simulink model "EngineControl_SLPV"  (R2016b)
settings: Solver=ode23tb  StartTime=0.0  StopTime=60  FixedStep=1e-3  MaxStep=1e-2  RelTol=0.001  EnableMultiTasking=on
values from neighbouring files (symbols this model uses):
  alpha = 0.1    [main_slpv.m]
  Ap = plt.a    [plant_sel.m]
  Bp = plt.b    [plant_sel.m]
  Cp = plt.c    [plant_sel.m]
  Dp = plt.d    [plant_sel.m]
  swtch = 1    [main_slpv.m]
  Wi = ss(tf([0.6 2],[1 0]))    [plant_sel.m]
undefined symbols (not defined in the file or in its folder): Khinf, sigbuilder_block
undefined symbols (not defined in the file): design_para, Dk, OptRst, theta_info
libraries: simulink x3
settings Model: Creator=Marius  LastModifiedBy=boran
settings DataIOCC: LimitDataPoints=on  SaveFormat=Array  SignalLoggingSaveFormat=ModelDataLogs
settings OptimizationCC: ExpressionDepthLimit=2147483647  InitFltsAndDblsToZero=on  LifeSpan=inf
settings DebuggingCC: UnderspecifiedInitializationDetection=Classic  MergeDetectMultiDrivingBlocksExec=none  SolverPrmCheckMsg=warning  FcnCallInpInsideContextMsg=warning  AllowSymbolicDim=off  StateNameClashWarn=warning  SFUnexpectedBacktrackingDiag=warning  SFNoUnconditionalDefaultTransitionDiag=warning  SFExecutionAtInitializationDiag=none
settings HardwareCC: ProdBitPerPointer=32  ProdBitPerSizeT=32  ProdBitPerPtrDiffT=32  ProdLargestAtomicFloat=None  ProdIntDivRoundTo=Undefined  ProdEndianess=Unspecified  ProdWordSize=32  ProdHWDeviceType=32-bit Generic
settings ModelReferenceCC: PropagateSignalLabelsOutOfModel=off
settings SFSimCC: SimParseCustomCode=off
settings GRTTargetCC: TargetLangStandard=C89/C90 (ANSI)  CombineOutputUpdateFcns=off  GRTInterface=on
settings ConfigComp: CovMetricSettings=dw  CovHtmlReporting=on  CovSaveCumulativeToWorkspaceVar=on  CovSaveSingleToWorkspaceVar=on  CovExternalEMLEnable=off  CovSFcnEnable=off

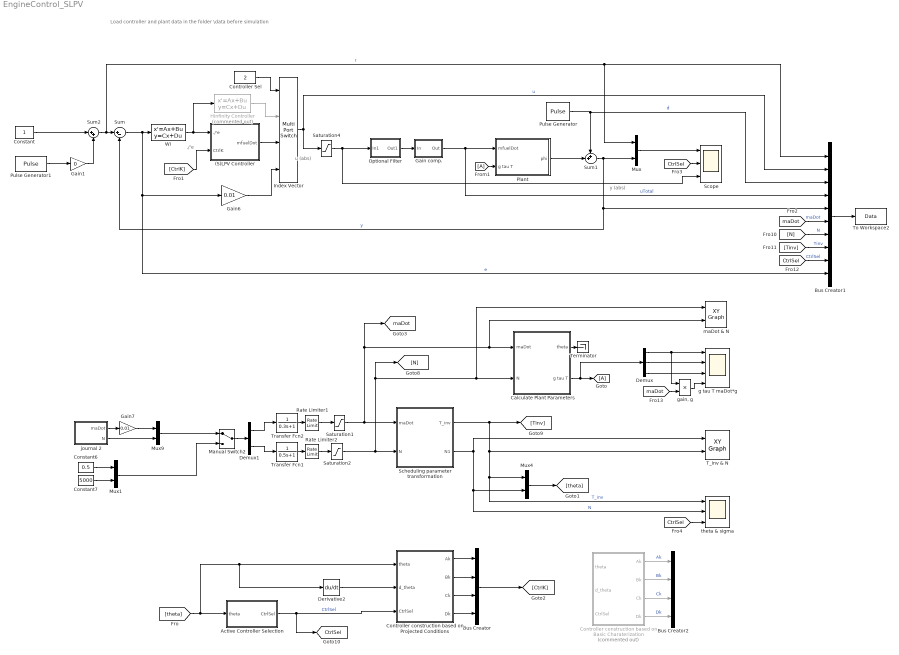
== system EngineControl_SLPV ==
  note: Load controller and plant data in the folder \data before simulation
  note: y (abs)
  note: u (abs)
  note: ./'e
  "(S)LPV Controller " : Subsystem
  Active Controller Selection : Subsystem
  Bus Creator : BusCreator  Inputs=4
  Bus Creator1 : BusCreator  Inputs=10
  Bus Creator2 : BusCreator  Inputs=4
  Calculate Plant Parameters : Subsystem
  Constant : Constant
  Constant6 : Constant  Value=0.5
  Constant7 : Constant  Value=5000
  Controller Sel : Constant  Value=2
  Controller construction based on Basic Charaterization : MATLAB Function  Commented=on  TreatAsAtomicUnit=on  mask{XY_PD=design_para.XY_PD, X=OptRst.X, Y=OptRst.Y, Ah=OptRst.K.Ah, Bh=OptRst.K.Bh, Ch=OptRst.K.Ch, Dh=OptRst.K.Dh, B2=0, C2=0}
  Controller construction based on Projected Conditions : MATLAB Function  TreatAsAtomicUnit=on  mask{XY_PD=design_para.XY_PD, X=OptRst.X, Y=OptRst.Y, Dk1=Dk, gam=OptRst.gam}
      mask prompts: Dk1 "Dk"
  Demux : Demux  Outputs=3
  Demux1 : Demux  Outputs=2
  Derivative2 : Derivative
  Gain comp. : Subsystem
  Gain1 : Gain  Gain=0
  Gain6 : Gain  Gain=0.01
  Gain7 : Gain  Gain=0.01
  Hinfinity Controller : StateSpace  Commented=on  A=Khinf.a  B=Khinf.b  C=Khinf.c  D=Khinf.d  X0=0
  Index Vector : MultiPortSwitch
  Manual Switch2 : ManualSwitch
  Mux{,1,4,9} (4 alike) : Mux  Inputs=2
  Optional Filter : Subsystem
  Plant : Subsystem
  Pulse Generator : DiscretePulseGenerator  PulseType=Time based  Amplitude=0.1  Period=20  PulseWidth=50
  Pulse Generator1 : DiscretePulseGenerator  PulseType=Time based  Amplitude=0.1  Period=20  PulseWidth=50
  Rate Limiter1 : RateLimiter
  Rate Limiter2 : RateLimiter  RisingSlewLimit=2000  FallingSlewLimit=-2000
  Saturation1 : Saturate  UpperLimit=1  LowerLimit=0.1  ZeroCross=off
  Saturation2 : Saturate  UpperLimit=6000  LowerLimit=800  ZeroCross=off
  Saturation4 : Saturate  UpperLimit=1  LowerLimit=0  ZeroCross=off
  Scheduling parameter transformation : Subsystem
  Scope : Scope  NumInputPorts=3
  Sum : Sum  Inputs=|+-
  Sum1 : Sum  Inputs=++|
  Sum2 : Sum  Inputs=|++
  T_inv & N : simulink/Sinks/XY Graph  xmin=0  xmax=6000  ymin=0  ymax=15  st=-1
  Terminator : Terminator
  To Workspace2 : ToWorkspace  VariableName=Data  SaveFormat=Timeseries  SampleTime=-1
  Transfer Fcn1 : TransferFcn  Denominator=[0.5 1]
  Transfer Fcn2 : TransferFcn  Denominator=[0.3 1]
  Wi : StateSpace  A=Wi.a  B=Wi.b  C=Wi.c  D=Wi.d  X0=0
  g tau T maDot*g : Scope  NumInputPorts=4
  "gain, g" : Product  RndMeth=Zero
  journal 2 : Subsystem  Tag=STV Subsys  LoadFcn=sigbuilder_block('load');  StartFcn=sigbuilder_block('start');  StopFcn=sigbuilder_block('stop');  ClipboardFcn=sigbuilder_block('clipboard');  mask(Sigbuilder block){tuvar=[0:10]}
      mask help: Sigbuilder GUI
      mask init:
      | if ~strcmp(get_param(bdroot(gcbh),'SimulationStatus'),'stopped') tuvar = sigbuilder_block('maskInit'); end
      settings: CopyFcn=sigbuilder_block('copy');  DeleteFcn=sigbuilder_block('delete');  ModelCloseFcn=sigbuilder_block('modelClose');  PreSaveFcn=sigbuilder_block('preSave');  PauseFcn=sigbuilder_block('pause')  ContinueFcn=sigbuilder_block('continue')  NameChangeFcn=sigbuilder_block('namechange');  OpenFcn=sigbuilder_block('open',[-1117.5 98.25 1428 499.5 ]);  CloseFcn=sigbuilder_block('close');
      mask Display: plot(0,0,100,100,[10,10,40,40,10],[80,20,20,80,80],[40,10],[50,50], [40,27,10],[65,72,56],[40,25,25,10],[28,28,43,43]);
  maDot & N : simulink/Sinks/XY Graph  xmin=0  xmax=6000  ymin=0  ymax=1  st=-1
  theta & sigma : Scope  NumInputPorts=3
  tag scope: CtrlSel=global, maDot=global
  wires:
  Mux/1 -> Scope/1
  Sum1/1 -> Mux/2, Bus Creator1/5, Sum/2  "y"
  Constant/1 -> Sum2/1
  Calculate Plant Parameters/1(theta) -> Terminator/1
  Demux/1 -> "gain, g"/1, g tau T maDot*g/1
  Demux/2 -> g tau T maDot*g/2
  Demux/3 -> g tau T maDot*g/3
  Calculate Plant Parameters/2(g tau T) -> [A], Demux/1
  [A] -> Plant/2(g tau T)
  Scheduling parameter transformation/2(N1) -> Mux4/2, theta & sigma/2, T_inv & N/1  "N"
  Scheduling parameter transformation/1(T_inv) -> T_inv & N/2, theta & sigma/1, Mux4/1, [Tinv]  "T_inv"
  Rate Limiter2/1 -> Saturation2/1
  Mux4/1 -> [theta]
  [theta] -> Derivative2/1, Controller construction based on Projected Conditions/1(theta), Active Controller Selection/1(theta)
  Controller construction based on Projected Conditions/3(Ck) -> Bus Creator/3
  Controller construction based on Projected Conditions/2(Bk) -> Bus Creator/2
  Controller construction based on Projected Conditions/4(Dk) -> Bus Creator/4
  Controller construction based on Projected Conditions/1(Ak) -> Bus Creator/1
  Active Controller Selection/1(CtrlSel) -> [CtrlSel], Controller construction based on Projected Conditions/3(CtrlSel)  "CtrlSel"
  Derivative2/1 -> Controller construction based on Projected Conditions/2(d_theta)
  Rate Limiter1/1 -> Saturation1/1
  Saturation1/1 -> Calculate Plant Parameters/1(maDot), maDot & N/2, [maDot], Scheduling parameter transformation/1(maDot)
  Mux1/1 -> Manual Switch2/2
  Plant/1(phi) -> Sum1/2
  Optional Filter/1(Out1) -> Gain comp./1(In)
  "(S)LPV Controller "/1(mfuelDot) -> Index Vector/3
  Hinfinity Controller/1 -> Index Vector/2
  Gain6/1 -> Index Vector/4
  Controller Sel/1 -> Index Vector/1
  Constant6/1 -> Mux1/1
  Constant7/1 -> Mux1/2
  Manual Switch2/1 -> Demux1/1
  Bus Creator1/1 -> To Workspace2/1
  Sum2/1 -> Sum/1, Mux/1, Bus Creator1/1  "r"
  Pulse Generator/1 -> Bus Creator1/3, Sum1/1  "d"
  Gain comp./1(Out) -> Bus Creator1/4, Plant/1(mfuelDot)  "uTotal"
  Index Vector/1 -> Saturation4/1, Bus Creator1/2  "u"
  [maDot] -> Bus Creator1/6  "maDot"
  [N] -> Bus Creator1/7  "N"
  [Tinv] -> Bus Creator1/8  "Tinv"
  [CtrlSel] -> Bus Creator1/9  "CtrlSel"
  Controller construction based on Basic Charaterization/1(Ak) -> Bus Creator2/1  "Ak"
  Controller construction based on Basic Charaterization/2(Bk) -> Bus Creator2/2  "Bk"
  Controller construction based on Basic Charaterization/3(Ck) -> Bus Creator2/3  "Ck"
  Controller construction based on Basic Charaterization/4(Dk) -> Bus Creator2/4  "Dk"
  [maDot] -> "gain, g"/2
  "gain, g"/1 -> g tau T maDot*g/4
  Bus Creator/1 -> [CtrlK]
  [CtrlK] -> "(S)LPV Controller "/2(CtrlK)
  Gain7/1 -> Mux9/1
  Mux9/1 -> Manual Switch2/1
  Saturation2/1 -> Calculate Plant Parameters/2(N), maDot & N/1, [N], Scheduling parameter transformation/2(N)
  Sum/1 -> Wi/1, Gain6/1, Bus Creator1/10  "e"
  Demux1/1 -> Transfer Fcn2/1
  Demux1/2 -> Transfer Fcn1/1
  Transfer Fcn2/1 -> Rate Limiter1/1
  Transfer Fcn1/1 -> Rate Limiter2/1
  journal 2/2(N) -> Mux9/2
  journal 2/1(maDot) -> Gain7/1
  Wi/1 -> "(S)LPV Controller "/1(./'e), Hinfinity Controller/1
  Saturation4/1 -> Optional Filter/1(In1), Scope/3
  Pulse Generator1/1 -> Gain1/1
  Gain1/1 -> Sum2/2
  [CtrlSel] -> Scope/2
  [CtrlSel] -> theta & sigma/3

== system EngineControl_SLPV/(S)LPV Controller  ==
  ./'e : Inport
  CtrlK : Inport  Port=2
  Controller2 : Subsystem
  Terminator1 : Terminator
  mfuelDot : Outport
  wires:
  Controller2/1(delta_u) -> mfuelDot/1
  Controller2/2(xk) -> Terminator1/1
  CtrlK/1 -> Controller2/2(CtrlK)
  ./'e/1 -> Controller2/1(./`e)

== system EngineControl_SLPV/Active Controller Selection ==
  theta : Inport
  Clock : Clock
  MATLAB Function2 : MATLAB Function  TreatAsAtomicUnit=on  mask{Theta1=theta_info.Theta1, Theta2=theta_info.Theta2, SwLogic=design_para.SwLogic, REGID=design_para.REGID}
  Memory1 : Memory  X0=1
  CtrlSel : Outport
  wires:
  theta/1 -> MATLAB Function2/1(theta)
  Memory1/1 -> MATLAB Function2/3(CtrlSel_t_1)
  MATLAB Function2/1(CtrlSel) -> CtrlSel/1, Memory1/1
  Clock/1 -> MATLAB Function2/2(time)

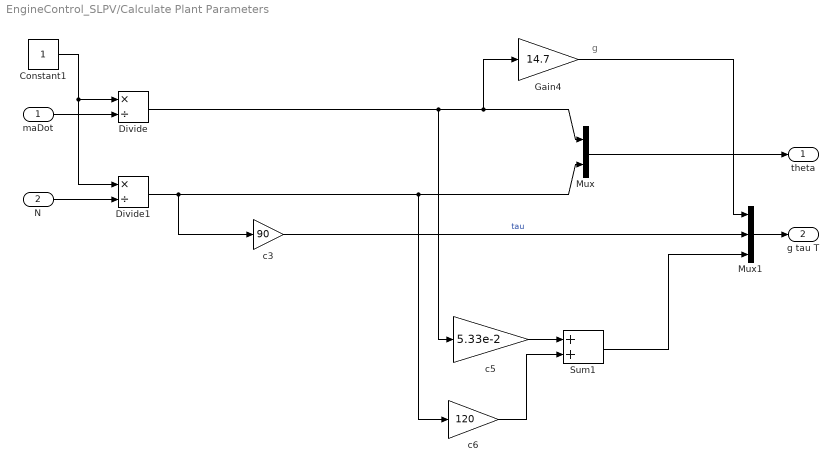
== system EngineControl_SLPV/Calculate Plant Parameters ==
  note: g
  maDot : Inport
  N : Inport  Port=2
  Constant1 : Constant
  Divide : Product  Inputs=*/
  Divide1 : Product  Inputs=*/
  Gain4 : Gain  Gain=14.7
  Mux : Mux  Inputs=2
  Mux1 : Mux  Inputs=3
  Sum1 : Sum
  c3 : Gain  Gain=90
  c5 : Gain  Gain=5.33e-2
  c6 : Gain  Gain=120
  theta : Outport
  g tau T : Outport  Port=2
  wires:
  Constant1/1 -> Divide/1, Divide1/1
  maDot/1 -> Divide/2
  N/1 -> Divide1/2
  Divide/1 -> c5/1, Gain4/1, Mux/1
  Divide1/1 -> c3/1, c6/1, Mux/2
  c6/1 -> Sum1/2
  c3/1 -> Mux1/2  "tau"
  Gain4/1 -> Mux1/1
  Mux/1 -> theta/1
  Mux1/1 -> g tau T/1
  c5/1 -> Sum1/1
  Sum1/1 -> Mux1/3

== system EngineControl_SLPV/Gain comp. ==
  In : Inport
  "gain, g" : Product  RndMeth=Zero
  Out : Outport
  wires:
  "gain, g"/1 -> Out/1
  [maDot] -> "gain, g"/2
  In/1 -> "gain, g"/1

== system EngineControl_SLPV/Optional Filter ==
  In1 : Inport
  Constant : Constant  Value=swtch+1
  Multiport Switch : MultiPortSwitch  Inputs=2
  Transfer Fcn : TransferFcn  Denominator=[alpha 1]
  Out1 : Outport
  wires:
  Multiport Switch/1 -> Out1/1
  In1/1 -> Transfer Fcn/1, Multiport Switch/2
  Transfer Fcn/1 -> Multiport Switch/3
  Constant/1 -> Multiport Switch/1

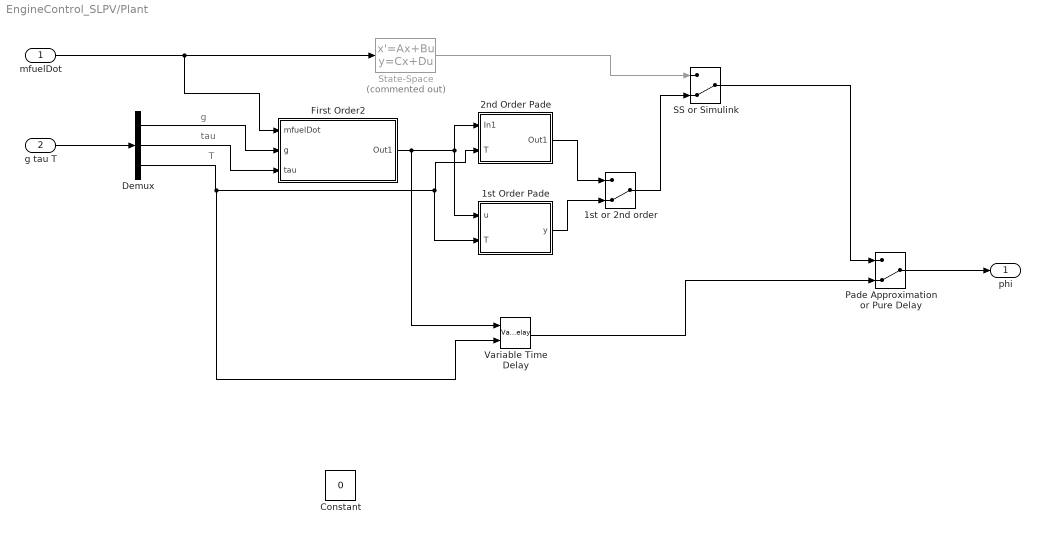
== system EngineControl_SLPV/Plant ==
  note: g
  note: tau
  note: T
  mfuelDot : Inport
  g tau T : Inport  Port=2
  1st Order Pade : Subsystem
  1st or 2nd order : ManualSwitch  CurrentSetting=0
  2nd Order Pade : Subsystem
  Constant : Constant  Value=0
  Demux : Demux  Outputs=3
  First Order2 : Subsystem
  Pade Approximation or Pure Delay : ManualSwitch  CurrentSetting=0
  SS or Simulink : ManualSwitch  CurrentSetting=0
  State-Space : StateSpace  Commented=on  A=Ap  B=Bp  C=Cp  D=Dp  X0=0
  Variable Time Delay : VariableTransportDelay  MaximumDelay=10  MaximumPoints=2048  ZeroDelay=on
  phi : Outport
  wires:
  Demux/1 -> First Order2/2(g)
  Demux/2 -> First Order2/3(tau)
  State-Space/1 -> SS or Simulink/1
  SS or Simulink/1 -> Pade Approximation or Pure Delay/1
  Pade Approximation or Pure Delay/1 -> phi/1
  g tau T/1 -> Demux/1
  2nd Order Pade/1(Out1) -> 1st or 2nd order/1
  1st Order Pade/1(y) -> 1st or 2nd order/2
  First Order2/1(Out1) -> Variable Time Delay/1, 2nd Order Pade/1(In1), 1st Order Pade/1(u)
  1st or 2nd order/1 -> SS or Simulink/2
  Variable Time Delay/1 -> Pade Approximation or Pure Delay/2
  mfuelDot/1 -> First Order2/1(mfuelDot), State-Space/1
  Demux/3 -> 2nd Order Pade/2(T), 1st Order Pade/2(T), Variable Time Delay/2

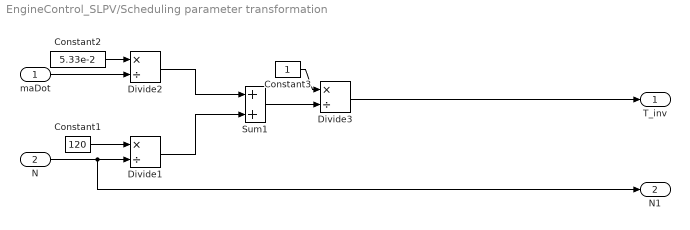
== system EngineControl_SLPV/Scheduling parameter transformation ==
  maDot : Inport
  N : Inport  Port=2
  Constant1 : Constant  Value=120
  Constant2 : Constant  Value=5.33e-2
  Constant3 : Constant
  Divide1 : Product  Inputs=*/
  Divide2 : Product  Inputs=*/
  Divide3 : Product  Inputs=*/
  Sum1 : Sum
  T_inv : Outport
  N1 : Outport  Port=2
  wires:
  N/1 -> N1/1, Divide1/2
  maDot/1 -> Divide2/2
  Constant1/1 -> Divide1/1
  Constant2/1 -> Divide2/1
  Divide2/1 -> Sum1/1
  Divide1/1 -> Sum1/2
  Sum1/1 -> Divide3/2
  Constant3/1 -> Divide3/1
  Divide3/1 -> T_inv/1

== system EngineControl_SLPV/journal 2 ==
  Demux : Demux  Tag=STV Demux  Outputs=2
  FromWs : FromWorkspace  Tag=STV FromWs  VariableName=tuvar  SampleTime=0
      SigBuilderData=|
      | common.afterFinalStr = 'Extrapolate'
      | common.sampleTime = 0
      | dataSet.timeRange = [0 90]
      | dataSet.name = 'Group 1'
      | sbobj.Groups.Name = 'Group 1'
      | sbobj.Groups.Signals(1).Name = 'maDot'
      | sbobj.Groups.Signals(1).XData = [0 3 5.6 8 10.9 14.8 19.7 22 24 26 27 30.8 32.5 33.5 35 36.2 38 39 39 41 41 43.4 45.5 47 48 52.3 54 56.5 59 60 65 65 70 90]
      | sbobj.Groups.Signals(1).YData = [10 10 13.6 13.5 19.1 38.6 39.1 26.6 29.1 65.1 97.6 98.6 98.6 40.6 40.6 96.6 97.1 97.1 97 96.5 97 45.1 81.1 82.1 40.1 40.6 63 38 33.5 33.5 35.5 40.1 39.1 8.5]
      | sbobj.Groups.Signals(2).Name = 'N'
      | sbobj.Groups.Signals(2).XData = [0 3 5.6 8 11.4 14 17 19.9 23 24 26.9 29 33.3 34.5 35.5 36.5 38 39 41 43.4 45.8 47.2 49 52 54 56.5 59 60 90]
      | sbobj.Groups.Signals(2).YData = [800 800 1000 800 1000 2050 5500 5500 2050 2000 2350 5750 5800 2620 2650 4850 4850 3700 3750 2750 3700 3700 2400 2400 3250 1800 1550 1550 1300]
      | sbobj.Groups.TimeRange = [0 90]
  maDot : Outport  Tag=STV Outport
  N : Outport  Tag=STV Outport  Port=2
  wires:
  FromWs/1 -> Demux/1
  Demux/1 -> maDot/1
  Demux/2 -> N/1

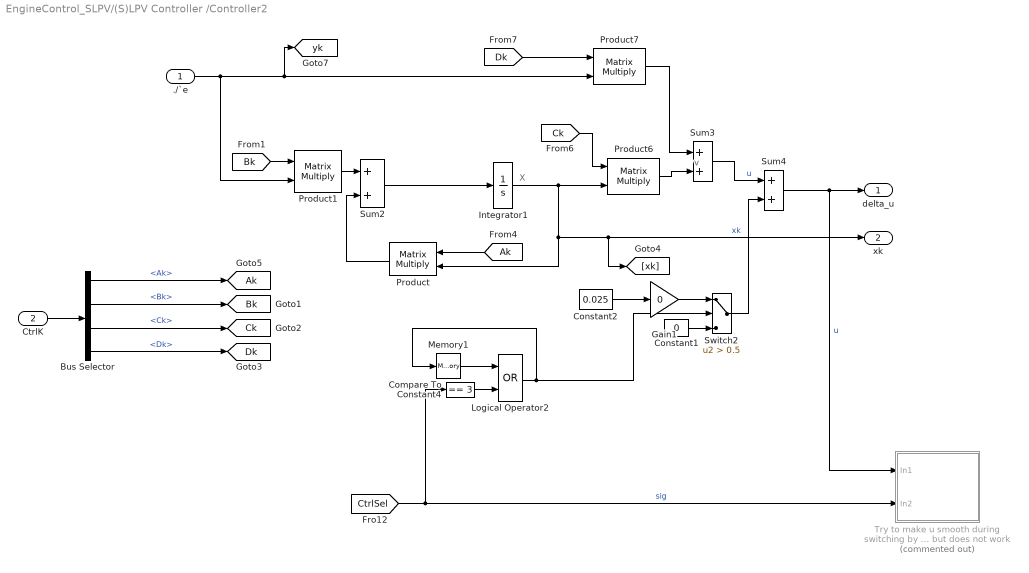
== system EngineControl_SLPV/(S)LPV Controller /Controller2 ==
  note: X
  note: v
  ./`e : Inport
  CtrlK : Inport  Port=2
  Bus Selector : BusSelector  OutputSignals=Ak,Bk,Ck,Dk
  Compare To Constant4 : simulink/Logic and Bit Operations/Compare To Constant  relop===  const=3  OutDataTypeStr=uint8
  Constant1 : Constant  Value=0
  Constant2 : Constant  Value=0.025  VectorParams1D=off
  Gain1 : Gain  Gain=0
  Integrator1 : Integrator
  Logical Operator2 : Logic  Operator=OR  AllPortsSameDT=off  OutDataTypeStr=boolean
  Memory1 : Memory
  Product{,1,6..7} (4 alike) : Product  Multiplication=Matrix(*)
  Sum2 : Sum
  Sum3 : Sum
  Sum4 : Sum
  Switch2 : Switch  Criteria=u2 > Threshold  Threshold=0.5
  Try to make u smooth during switching by resetting controller state but does not work : Subsystem  Commented=on
  delta_u : Outport
  xk : Outport  Port=2
  tag scope: Ak=global, Bk=global, Ck=global, Dk=global, yk=global
  wires:
  Sum4/1 -> Try to make u smooth during switching by resetting controller state but does not work/1(In1), delta_u/1  "u"
  [CtrlSel] -> Try to make u smooth during switching by resetting controller state but does not work/2(In2), Compare To Constant4/1  "sig"
  Product6/1 -> Sum3/2
  Product1/1 -> Sum2/1
  [Bk] -> Product1/1
  Product/1 -> Sum2/2
  [Ak] -> Product/1
  Bus Selector/4 -> [Dk]  "<Dk>"
  Bus Selector/3 -> [Ck]  "<Ck>"
  Bus Selector/2 -> [Bk]  "<Bk>"
  Bus Selector/1 -> [Ak]  "<Ak>"
  [Ck] -> Product6/1
  [Dk] -> Product7/1
  Product7/1 -> Sum3/1
  ./`e/1 -> Product1/2, Product7/2, [yk]
  Integrator1/1 -> Product/2, [xk], xk/1, Product6/2  "xk"
  Sum2/1 -> Integrator1/1
  CtrlK/1 -> Bus Selector/1
  Constant1/1 -> Switch2/3
  Logical Operator2/1 -> Switch2/2, Memory1/1
  Sum3/1 -> Sum4/1  "u"
  Switch2/1 -> Sum4/2
  Constant2/1 -> Gain1/1
  Compare To Constant4/1 -> Logical Operator2/2
  Memory1/1 -> Logical Operator2/1
  Gain1/1 -> Switch2/1

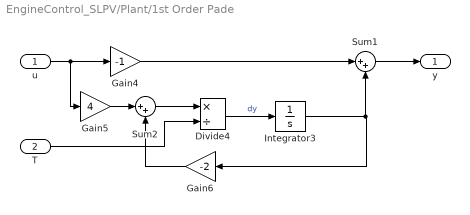
== system EngineControl_SLPV/Plant/1st Order Pade ==
  u : Inport
  T : Inport  Port=2
  Divide4 : Product  Inputs=*/
  Gain4 : Gain  Gain=-1
  Gain5 : Gain  Gain=4
  Gain6 : Gain  Gain=-2
  Integrator3 : Integrator
  Sum1 : Sum  Inputs=|++
  Sum2 : Sum  Inputs=|++
  y : Outport
  wires:
  u/1 -> Gain5/1, Gain4/1
  Integrator3/1 -> Gain6/1, Sum1/2
  Divide4/1 -> Integrator3/1  "dy"
  Gain5/1 -> Sum2/1
  Gain6/1 -> Sum2/2
  Sum2/1 -> Divide4/1
  T/1 -> Divide4/2
  Gain4/1 -> Sum1/1
  Sum1/1 -> y/1

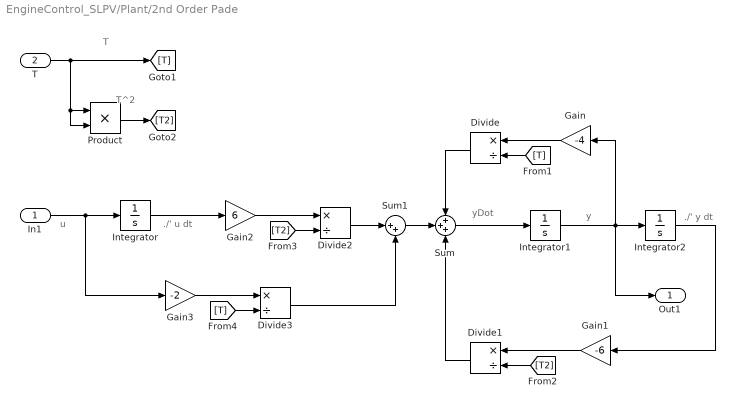
== system EngineControl_SLPV/Plant/2nd Order Pade ==
  note: u
  note: ./' u dt
  note: yDot
  note: y
  note: ./' y dt
  note: T
  note: T^2
  In1 : Inport
  T : Inport  Port=2
  Divide{,1..3} (4 alike) : Product  Inputs=*/
  Gain : Gain  Gain=-4
  Gain1 : Gain  Gain=-6
  Gain2 : Gain  Gain=6
  Gain3 : Gain  Gain=-2
  Integrator : Integrator
  Integrator1 : Integrator
  Integrator2 : Integrator
  Product : Product  RndMeth=Zero
  Sum : Sum  Inputs=+++
  Sum1 : Sum  Inputs=|++
  Out1 : Outport
  wires:
  In1/1 -> Integrator/1, Gain3/1
  Integrator/1 -> Gain2/1
  Integrator1/1 -> Integrator2/1, Gain/1, Out1/1
  Sum/1 -> Integrator1/1
  Sum1/1 -> Sum/2
  T/1 -> Product/1, Product/2, [T]
  Gain/1 -> Divide/1
  Divide/1 -> Sum/1
  Gain1/1 -> Divide1/1
  Integrator2/1 -> Gain1/1
  Divide1/1 -> Sum/3
  Product/1 -> [T2]
  [T] -> Divide/2
  [T2] -> Divide1/2
  Gain2/1 -> Divide2/1
  [T2] -> Divide2/2
  Divide2/1 -> Sum1/1
  Gain3/1 -> Divide3/1
  [T] -> Divide3/2
  Divide3/1 -> Sum1/2

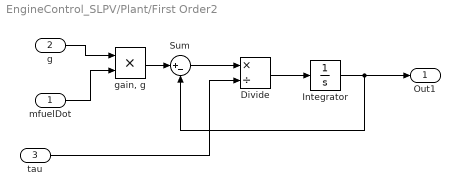
== system EngineControl_SLPV/Plant/First Order2 ==
  mfuelDot : Inport
  g : Inport  Port=2
  tau : Inport  Port=3
  Divide : Product  Inputs=*/
  Integrator : Integrator
  Sum : Sum  Inputs=|+-
  "gain, g" : Product  RndMeth=Zero
  Out1 : Outport
  wires:
  "gain, g"/1 -> Sum/1
  Sum/1 -> Divide/1
  Divide/1 -> Integrator/1
  mfuelDot/1 -> "gain, g"/2
  g/1 -> "gain, g"/1
  tau/1 -> Divide/2
  Integrator/1 -> Out1/1, Sum/2

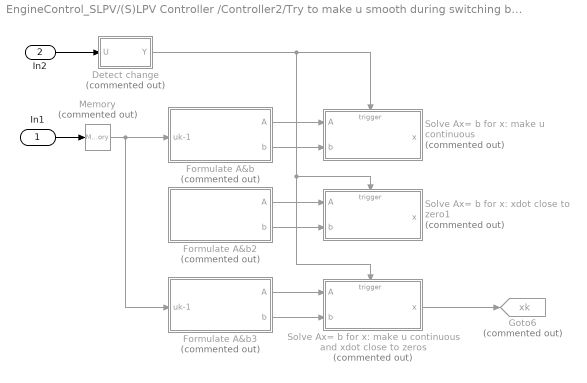
== system EngineControl_SLPV/(S)LPV Controller /Controller2/Try to make u smooth during switching by resetting controller state but does not work ==
  In1 : Inport
  In2 : Inport  Port=2
  "Detect change " : Subsystem  Commented=on
  Formulate A&b : Subsystem  Commented=on
  Formulate A&b2 : Subsystem  Commented=on
  Formulate A&b3 : Subsystem  Commented=on
  Goto6 : Goto  Commented=on  GotoTag=xk  TagVisibility=global
  Memory : Memory  Commented=on
  Solve Ax= b for x: xdot close to zero1 : Subsystem  Commented=on  TreatAsAtomicUnit=on
  "Solve Ax= b for x: make u continuous " : Subsystem  Commented=on  TreatAsAtomicUnit=on
  "Solve Ax= b for x: make u continuous and xdot close to zeros " : Subsystem  Commented=on  TreatAsAtomicUnit=on
  wires:
  In1/1 -> Memory/1
  In2/1 -> "Detect change "/1(U)
  Formulate A&b/1(A) -> "Solve Ax= b for x: make u continuous "/1(A)
  Formulate A&b/2(b) -> "Solve Ax= b for x: make u continuous "/2(b)
  Formulate A&b2/1(A) -> Solve Ax= b for x: xdot close to zero1/1(A)
  Formulate A&b2/2(b) -> Solve Ax= b for x: xdot close to zero1/2(b)
  "Solve Ax= b for x: make u continuous and xdot close to zeros "/1(x) -> Goto6/1
  Formulate A&b3/1(A) -> "Solve Ax= b for x: make u continuous and xdot close to zeros "/1(A)
  Formulate A&b3/2(b) -> "Solve Ax= b for x: make u continuous and xdot close to zeros "/2(b)
  Memory/1 -> Formulate A&b3/1(uk-1), Formulate A&b/1(uk-1)
  "Detect change "/1(Y) -> "Solve Ax= b for x: make u continuous and xdot close to zeros "/Trigger, Solve Ax= b for x: xdot close to zero1/Trigger, "Solve Ax= b for x: make u continuous "/Trigger

== system EngineControl_SLPV/(S)LPV Controller /Controller2/Try to make u smooth during switching by resetting controller state but does not work/Detect change  ==
  note: U(k)
  note: Edge
  U : Inport
  FixPt Relational Operator : RelationalOperator  Operator=~=  OutDataTypeStr=boolean  ZeroCross=off  RndMeth=Nearest
  Memory : Memory
  Y : Outport  InitialOutput=0
  wires:
  U/1 -> FixPt Relational Operator/1, Memory/1
  FixPt Relational Operator/1 -> Y/1
  Memory/1 -> FixPt Relational Operator/2  "U(k-1)"

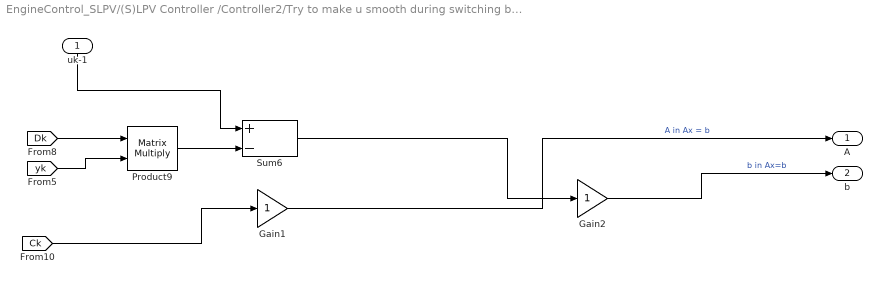
== system EngineControl_SLPV/(S)LPV Controller /Controller2/Try to make u smooth during switching by resetting controller state but does not work/Formulate A&b ==
  uk-1 : Inport
  Gain1 : Gain
  Gain2 : Gain
  Product9 : Product  Multiplication=Matrix(*)
  Sum6 : Sum  Inputs=+-
  A : Outport
  b : Outport  Port=2
  wires:
  [yk] -> Product9/2
  uk-1/1 -> Sum6/1
  [Dk] -> Product9/1
  Sum6/1 -> Gain2/1
  Product9/1 -> Sum6/2
  [Ck] -> Gain1/1
  Gain2/1 -> b/1  "b in Ax=b"
  Gain1/1 -> A/1  "A in Ax = b"

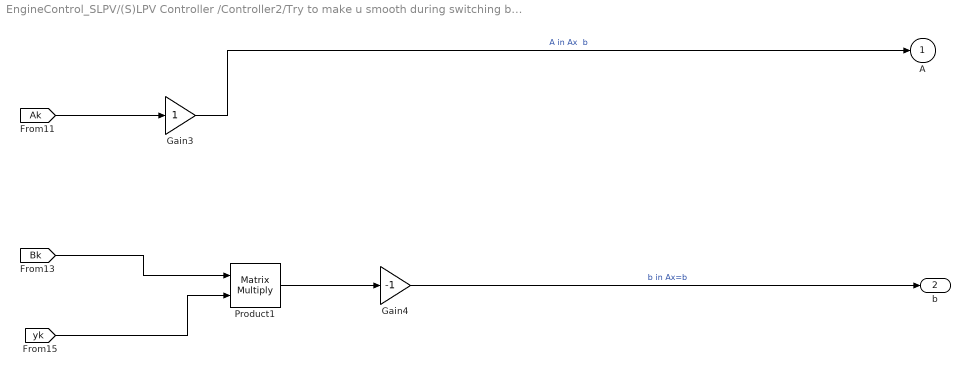
== system EngineControl_SLPV/(S)LPV Controller /Controller2/Try to make u smooth during switching by resetting controller state but does not work/Formulate A&b2 ==
  Gain3 : Gain
  Gain4 : Gain  Gain=-1
  Product1 : Product  Multiplication=Matrix(*)
  A : Outport
  b : Outport  Port=2
  wires:
  Product1/1 -> Gain4/1
  [yk] -> Product1/2
  [Ak] -> Gain3/1
  [Bk] -> Product1/1
  Gain3/1 -> A/1  "A in Ax  b"
  Gain4/1 -> b/1  "b in Ax=b"

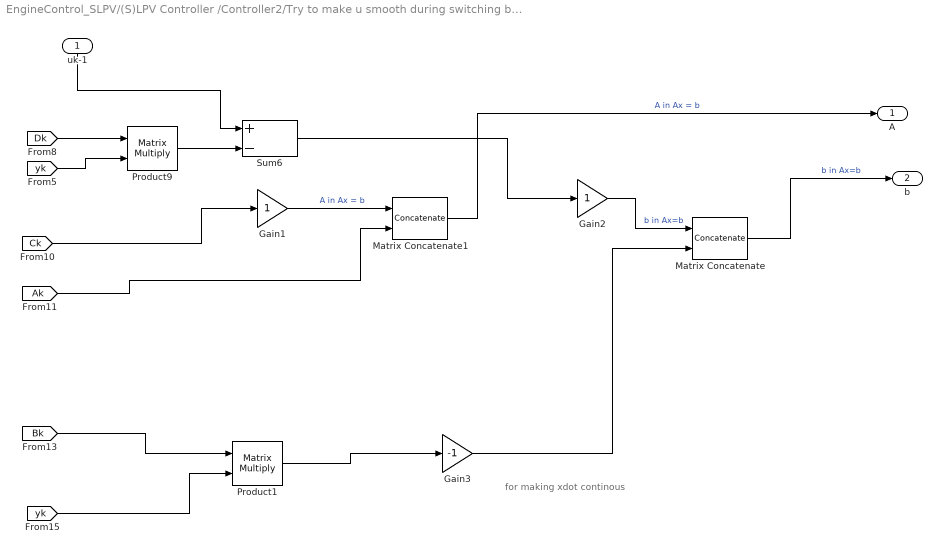
== system EngineControl_SLPV/(S)LPV Controller /Controller2/Try to make u smooth during switching by resetting controller state but does not work/Formulate A&b3 ==
  note: for making xdot continous
  uk-1 : Inport
  Gain1 : Gain
  Gain2 : Gain
  Gain3 : Gain  Gain=-1
  Matrix Concatenate : Concatenate  Mode=Multidimensional array
  Matrix Concatenate1 : Concatenate  Mode=Multidimensional array
  Product1 : Product  Multiplication=Matrix(*)
  Product9 : Product  Multiplication=Matrix(*)
  Sum6 : Sum  Inputs=+-
  A : Outport
  b : Outport  Port=2
  wires:
  [yk] -> Product9/2
  uk-1/1 -> Sum6/1
  [Dk] -> Product9/1
  Sum6/1 -> Gain2/1
  Product9/1 -> Sum6/2
  [Bk] -> Product1/1
  [Ck] -> Gain1/1
  [yk] -> Product1/2
  Product1/1 -> Gain3/1
  [Ak] -> Matrix Concatenate1/2
  Gain3/1 -> Matrix Concatenate/2
  Gain1/1 -> Matrix Concatenate1/1  "A in Ax = b"
  Gain2/1 -> Matrix Concatenate/1  "b in Ax=b"
  Matrix Concatenate1/1 -> A/1  "A in Ax = b"
  Matrix Concatenate/1 -> b/1  "b in Ax=b"

== system EngineControl_SLPV/(S)LPV Controller /Controller2/Try to make u smooth during switching by resetting controller state but does not work/Solve Ax= b for x: xdot close to zero1 ==
  A : Inport
  b : Inport  Port=2
  Trigger : TriggerPort  VariantControl=Variant
  Divide : Product  Inputs=**  Multiplication=Matrix(*)
  Pseudo Inverse for full row-rank mat : Subsystem
  x : Outport
  wires:
  Divide/1 -> x/1
  b/1 -> Divide/2
  A/1 -> Pseudo Inverse for full row-rank mat/1(A)
  Pseudo Inverse for full row-rank mat/1(A*(AA*)^-1) -> Divide/1

== system EngineControl_SLPV/(S)LPV Controller /Controller2/Try to make u smooth during switching by resetting controller state but does not work/Solve Ax= b for x: make u continuous  ==
  A : Inport
  b : Inport  Port=2
  Trigger : TriggerPort  VariantControl=Variant
  Divide : Product  Inputs=**  Multiplication=Matrix(*)
  Pseudo Inverse for full row-rank mat : Subsystem
  x : Outport
  wires:
  Pseudo Inverse for full row-rank mat/1(A*(AA*)^-1) -> Divide/1
  A/1 -> Pseudo Inverse for full row-rank mat/1(A)
  b/1 -> Divide/2
  Divide/1 -> x/1

== system EngineControl_SLPV/(S)LPV Controller /Controller2/Try to make u smooth during switching by resetting controller state but does not work/Solve Ax= b for x: make u continuous and xdot close to zeros  ==
  A : Inport
  b : Inport  Port=2
  Trigger : TriggerPort  VariantControl=Variant
  Divide : Product  Inputs=**  Multiplication=Matrix(*)
  Pseudo Inverse for full row-rank mat : Subsystem
  x : Outport
  wires:
  Pseudo Inverse for full row-rank mat/1(A*(AA*)^-1) -> Divide/1
  A/1 -> Pseudo Inverse for full row-rank mat/1(A)
  b/1 -> Divide/2
  Divide/1 -> x/1

== system EngineControl_SLPV/(S)LPV Controller /Controller2/Try to make u smooth during switching by resetting controller state but does not work/Solve Ax= b for x: xdot close to zero1/Pseudo Inverse for full row-rank mat ==
  A : Inport
  Divide1 : Product  Inputs=**  Multiplication=Matrix(*)
  Divide2 : Product  Inputs=/  Multiplication=Matrix(*)
  Divide3 : Product  Inputs=**  Multiplication=Matrix(*)
  Math Function : Math  Operator=transpose  SaturateOnIntegerOverflow=on
  A*(AA*)^-1 : Outport
  wires:
  Divide2/1 -> Divide3/2
  A/1 -> Divide1/1, Math Function/1
  Divide3/1 -> A*(AA*)^-1/1
  Divide1/1 -> Divide2/1
  Math Function/1 -> Divide3/1, Divide1/2

== system EngineControl_SLPV/(S)LPV Controller /Controller2/Try to make u smooth during switching by resetting controller state but does not work/Solve Ax= b for x: make u continuous /Pseudo Inverse for full row-rank mat ==
  A : Inport
  Divide1 : Product  Inputs=**  Multiplication=Matrix(*)
  Divide2 : Product  Inputs=/  Multiplication=Matrix(*)
  Divide3 : Product  Inputs=**  Multiplication=Matrix(*)
  Math Function : Math  Operator=transpose  SaturateOnIntegerOverflow=on
  A*(AA*)^-1 : Outport
  wires:
  Math Function/1 -> Divide1/2, Divide3/1
  Divide1/1 -> Divide2/1
  Divide3/1 -> A*(AA*)^-1/1
  A/1 -> Math Function/1, Divide1/1
  Divide2/1 -> Divide3/2

== system EngineControl_SLPV/(S)LPV Controller /Controller2/Try to make u smooth during switching by resetting controller state but does not work/Solve Ax= b for x: make u continuous and xdot close to zeros /Pseudo Inverse for full row-rank mat ==
  A : Inport
  Divide1 : Product  Inputs=**  Multiplication=Matrix(*)
  Divide2 : Product  Inputs=/  Multiplication=Matrix(*)
  Divide3 : Product  Inputs=**  Multiplication=Matrix(*)
  Math Function : Math  Operator=transpose  SaturateOnIntegerOverflow=on
  A*(AA*)^-1 : Outport
  wires:
  Math Function/1 -> Divide1/2, Divide3/1
  Divide1/1 -> Divide2/1
  Divide3/1 -> A*(AA*)^-1/1
  A/1 -> Math Function/1, Divide1/1
  Divide2/1 -> Divide3/2

== matlab function EngineControl_SLPV/Active Controller Selection/MATLAB Function2 ==
  data: theta input; time input; CtrlSel output; CtrlSel_t_1 input; Theta1 parameter; Theta2 parameter; SwLogic parameter; REGID parameter
% function [Ak1,Bk1,Ck1,Dk1,Ak2,Bk2,Ck2,Dk2,Ak_a,Bk_a,Ck_a,Dk_a,CtrlSel]  = Controller(theta,time,CtrlSel_t_1,A_0,...
%     A_1,A_2,B2,C2,XZ_PD,X,Z,Ah,Bh,Ch,Dh,reg)
function CtrlSel   = Controller(theta,time,CtrlSel_t_1,Theta1,Theta2,SwLogic,REGID)
if CtrlSel_t_1 >REGID(end,1)
    CtrlSel_t_1 = REGID(end,1);
end
regid = REGID(CtrlSel_t_1,2:3);
Theta1N = ones(4,2)*NaN;
Theta2N = ones(4,2)*NaN;
Theta1N(1:size(Theta1,1),:) = Theta1;
Theta2N(1:size(Theta2,1),:) = Theta2;
if SwLogic == 0
    CtrlSel = 1;
else
    if (time==0)
    %     display('Simulation starts');
        if theta(1) > Theta1N(4,1)
            regid(1) = 4;
        elseif theta(1) > Theta1N(3,1) && theta(1) < Theta1N(3,2)
            regid(1) = 3;        
        elseif theta(1) > Theta1N(2,1) && theta(1) < Theta1N(2,2)  %subset 2
            regid(1) = 2;
        elseif theta(1) < Theta1N(1,2) % 1
                regid(1) = 1; 
        end
        if theta(2) < Theta2N(1,2) %subset 1
            regid(2) = 1;
        elseif theta(2) > Theta2N(2,1) && theta(2) < Theta2N(2,2) %subset 2
            regid(2) = 2;
        elseif theta(2) > Theta2N(3,1)
            regid(2) = 3;
        end
    else
        switch regid(1)
            case 1
                if  theta(1) > Theta1N(1,2) %subset 2
                    regid(1) = 2;
                end
            case 2
                if theta(1) < Theta1N(2,1) %subset 1
                    regid(1) = 1;
                elseif theta(1) > Theta1N(2,2)
                    regid(1) = 3;
                end
            case 3
                if theta(1) < Theta1N(3,1)
                    regid(1) = 2;
                elseif theta(1) > Theta1N(3,2)
                    regid(1) = 4;
                end
            case 4
                 if theta(1) < Theta1N(4,1)
                    regid(1) = 3;
                 end                
        end
        
        switch regid(2)
            case 1
                if  theta(2) > Theta2N(1,2) %subset 2
                    regid(2) = 2;
                end
            case 2
                if theta(2) < Theta2N(2,1) %subset 1
                    regid(2) = 1;
                elseif theta(2) > Theta2N(2,2)
                    regid(2) = 3;
                end
            case 3
                if theta(2) < Theta2N(3,1)
                    regid(2) = 2;
                end
        end       
    end
    CtrlSel = (regid(2)-1)*2 + regid(1);
end

== matlab function EngineControl_SLPV/Controller construction based on Projected Conditions ==
  data: Ak output; Bk output; Ck output; Dk output; theta input; d_theta input; CtrlSel input; XY_PD parameter; X parameter; Y parameter; Dk1 parameter; gam parameter
function [Ak,Bk,Ck,Dk]  = CtrlConstr(theta,d_theta,CtrlSel,XY_PD,X,Y,Dk1,gam)
regid = CtrlSel;
regnum = length(gam);
if regid>= regnum % for test
    regid = regnum; % regid may be larger than regnum when the solver step size is set to auto
end
Dk = Dk1(:,:,regid);
n = size(X,1);
In = eye(n);
XdYplusNdM = zeros(n);
X_t = zeros(n);
Y_t = zeros(n);
M = zeros(n);
N = zeros(n);
% if XY_PD == 2
%     Y_t = Y(:,:,1,regid)+theta(1)*Y(:,:,2,regid)+theta(2)*Y(:,:,3,regid);
%     X_t = X(:,:,1);
%     M = Y_t-In/X_t;
%     N = -X_t;    
% end
% if XY_PD == 1
%     Y_t = Y(:,:,1,regid);
%     X_t = X(:,:,1,regid)+theta(1)*X(:,:,2,regid)+theta(2)*X(:,:,3,regid); 
%     M = -Y_t;
%     N = X_t-In/Y_t;
% end
if XY_PD == 3
    Y_t = Y(:,:,1,regid)+theta(1)*Y(:,:,2,regid)+theta(2)*Y(:,:,3,regid);
    X_t = X(:,:,1,regid)+theta(1)*X(:,:,2,regid)+theta(2)*X(:,:,3,regid); 
    M = -Y_t;
    N = X_t-In/Y_t;  
    dY = d_theta(1)*Y(:,:,2,regid)+d_theta(2)*Y(:,:,3,regid);
    XdYplusNdM = Y_t\dY;
    % X*dY + N*dM = Y^-1*dY;
end    

%% First way
num_gain = 1;
ncyl = 4;
tau = 2*60*(ncyl-1)/ncyl/(theta(2)*num_gain);
Rstoich = 14.7;
g = Rstoich; % 
%     Tinv = 1./(120./theta(2)+ c./ma);
%% first order pade approximation of pure delay
Ap = [-1/tau 4*g*theta(1); 0 -2*theta(1)];
Bp = [-g 1].';
Cp = [1/tau 0];    
Dp = 0;    

 
%     Cp*inv(s*eye(length(Ap))-Ap)*Bp
np = size(Ap,1);

%     coder.extrinsic('tf','ss');
Wi.a = 0;
Wi.b = 2;
Wi.c = 1;
Wi.d = 0.6;

np = size(Ap,1);     
%% weigthting function 
We = 1;nwe = 0;
Wu = 1e1; nwu = 0;
nint = 1; % order of integrator  

A = [Ap, zeros(np,nwe+nwu+nint);...           
    -Wi.b*Cp, zeros(nint,nwe+nwu) Wi.a];
B1 =  [zeros(np,2);...
    -Wi.b, Wi.b];
B2 = [Bp;-Wi.b*Dp];
C1 = [[-Wi.d*Cp zeros(1,nwe+nwu), Wi.c]*We;...
    zeros(1,np+nwe), zeros(1,nint)];
D11 = [-We*Wi.d, We*Wi.d;...
    zeros(1,2)];
D12 = [-We*Wi.d*Dp; Wu];
C2 = [-Wi.d*Cp zeros(1,nwe+nwu), Wi.c];  
D21 = [-Wi.d Wi.d];
D22 = -Wi.d*Dp;


ny = size(D21,1);ny=ny(1);
nu = size(B2,2);nu=nu(1);
nw = size(B1,2); %nu = size(Gasym.B2,2);
nz = size(C1,1); %ny = size(Gasym.C2,1); 

Dcl = D11+D12*Dk*D21;
% Solve for Bkh and Ckh

TmpB  = linsolve([zeros(ny) D21 zeros(ny,nz); D21' -gam(regid)*eye(nw) Dcl'; zeros(nz,ny) Dcl -gam(regid)*eye(nz)]...
    ,-[C2;B1'*X_t;C1+D12*Dk*C2]);
TmpC = linsolve([zeros(nu) D12' zeros(nu,nw); D12 -gam(regid)*eye(nz) Dcl; zeros(nw,nu) Dcl' -gam(regid)*eye(nw)]...
    ,-[B2';C1*Y_t;(B1+B2*Dk*D21)']);
Bkh = TmpB(1:ny,:)';  Ckh = TmpC(1:nu,:);

% compute Akh
Akh = -(A+B2*Dk*C2)'+[X_t*B1+Bkh*D21 (C1+D12*Dk*C2)']/[-gam(regid)*eye(nw) Dcl';Dcl -gam(regid)*eye(nz)]*...
    [(B1+B2*Dk*D21)';C1*Y_t+D12*Ckh];

% compute Ak,Bk,Ck
Ninv = N\In;
Minv = In/M;

Ak = Ninv*(XdYplusNdM+Akh-X_t*(A-B2*Dk*C2)*Y_t-Bkh*C2*Y_t-X_t*B2*Ckh)*Minv';
Bk = Ninv*(Bkh-X_t*B2*Dk);
Ck = (Ckh-Dk*C2*Y_t)*Minv';

% Dk(:,:,regid) = Dh_t(:,:,regid);
% Ck(:,:,regid) = (Ch_t(:,:,regid) - Dk(:,:,regid)*C2*X_t(:,:,regid))/M(:,:,regid)';
% Bk(:,:,regid) = N(:,:,regid)\(Bh_t(:,:,regid)-Y_t(:,:,regid)*B2*Dk(:,:,regid));
% Ak(:,:,regid) =  N(:,:,regid)\(Ah_t(:,:,regid)-Bh_t(:,:,regid)*C2*X_t(:,:,regid)-...
%     Y_t(:,:,regid)*B2*Ch_t(:,:,regid)-Y_t(:,:,regid)*(A_t-B2*Dh_t(:,:,regid)*C2)*X_t(:,:,regid))/M(:,:,regid)';    


%     if XY_PD == 0
%         X_t  = X(:,:,1);
%         Y_t  = Y(:,:,1);
%         M  = -X_t;
%         N =  Y_t - eye(n)/X_t;
%     else
%         X_t  = X(:,:,regid);
%         Y_t  = Y(:,:,regid);
%         M  = -X_t;
%         N =  Y_t - eye(n)/X_t;
%     end
%     
   
%     if XY_PD == 1
%         X_t = X(:,:,1,regid)+theta(1)*X(:,:,2,regid)+theta(2)*X(:,:,3,regid);
%         Y_t = Y(:,:,1);
%         N = -Y_t;
%         M = X_t - eye(n)/Y_t;       
%     else
%         X_t = X(:,:,1);
%         Y_t = Y(:,:,1);
%         M = -X_t;
%         N =  Y_t - eye(n)/X_t;       
%     end
%     Dk_a = Dh_t ;
%     Ck_a = (Ch_t - Dk_a*C2*X_t)/M';
%     Bk_a = N\(Bh_t -Y_t*B2*Dk_a);
%     Ak_a =  N\(Ah_t -Bh_t*C2*X_t -...
%         Y_t*B2*Ch_t -Y_t*(A_t-B2*Dh_t*C2)*X_t)/M';    
%     if SwLogic == 2 % for average dwell time switching
%         Ak_a = Ak_a + lambda0/2*eye(n);
%     end
% end

== matlab function EngineControl_SLPV/Controller construction based on Basic Charaterization ==
  data: Ak output; Bk output; Ck output; Dk output; theta input; d_theta input; CtrlSel input; B2 parameter; C2 parameter; XY_PD parameter; X parameter; Y parameter; Ah parameter; Bh parameter; Ch parameter; Dh parameter
function [Ak,Bk,Ck,Dk]  = Controller(theta,d_theta,CtrlSel,B2,C2,XY_PD,X,Y,Ah,Bh,Ch,Dh)
regid = CtrlSel;
% plant 
n = size(X,1);
In = eye(n);
% first order pade approximation
A = [ -theta(2)/90, (294*theta(1))/5, 0;...
    0, -2*theta(1), 0;...
    -theta(2)/45, 0, 0];
B2 = [-14.7000,1.0000,0]';
C2 = [-theta(2)/150, 0, 1];

% second order pade approximation
% A = [-theta(2)/90,  6*theta(1)^2, -2*theta(1), 0;
%     0,           0,         1, 0;
%     0, -6*theta(1)^2, -4*theta(1), 0;
%     -(49*theta(2))/150,           0,         0, 0];
% B2 = [0 0 1 0]';
% C2 = [ -(49*theta(2))/500, 0, 0, 1];
XdYplusNdM = zeros(n);
X_t = zeros(n);
Y_t = zeros(n);
M = zeros(n);
N = zeros(n);
if XY_PD == 2
    Y_t = Y(:,:,1,regid)+theta(1)*Y(:,:,2,regid)+theta(2)*Y(:,:,3,regid);
    X_t = X(:,:,1);
    M = Y_t-In/X_t;
    N = -X_t;    
end
% if XY_PD == 1
%     Y_t = Y(:,:,1,regid);
%     X_t = X(:,:,1,regid)+theta(1)*X(:,:,2,regid)+theta(2)*X(:,:,3,regid); 
%     M = -Y_t;
%     N = X_t-In/Y_t;
% end
% if XY_PD == 3
%     Y_t = Y(:,:,1,regid)+theta(1)*Y(:,:,2,regid)+theta(2)*Y(:,:,3,regid);
%     X_t = X(:,:,1,regid)+theta(1)*X(:,:,2,regid)+theta(2)*X(:,:,3,regid); 
%     M = -Y_t;
%     N = X_t-In/Y_t;  
%     dY = d_theta(1)*Y(:,:,2,regid)+d_theta(2)*Y(:,:,3,regid);
%     XdYplusNdM = Y_t\dY;
%     % X*dY + N*dM = Y^-1*dY;
% end 

Akh = Ah(:,:,1,regid)+theta(1)*Ah(:,:,2,regid)+theta(2)*Ah(:,:,3,regid);
Bkh = Bh(:,:,1,regid)+theta(1)*Bh(:,:,2,regid)+theta(2)*Bh(:,:,3,regid);
Ckh = Ch(:,:,1,regid)+theta(1)*Ch(:,:,2,regid)+theta(2)*Ch(:,:,3,regid);
Dk = Dh(:,:,1,regid)+theta(1)*Dh(:,:,2,regid)+theta(2)*Dh(:,:,3,regid);

% compute Ak,Bk,Ck
Ninv = N\In;
Minv = In/M;

Ak = Ninv*(XdYplusNdM+Akh-X_t*(A-B2*Dk*C2)*Y_t-Bkh*C2*Y_t-X_t*B2*Ckh)*Minv';
Bk = Ninv*(Bkh-X_t*B2*Dk);
Ck = (Ckh-Dk*C2*Y_t)*Minv';
end
